simulink subsystem "PvtSubSys_VSM_ALL"  (R2020b)
settings: Solver=VariableStepAuto  StartTime=0.0  StopTime=10.0  RelTol=1e-3
values from neighbouring files (symbols this model uses):
  P_VSM_NOH_Act_Req = 0    [VSM_All.sldd]
  P_VSM_NOH_Swt_Req = 0    [VSM_All.sldd]
undefined symbols (not defined in the file or in its folder): ACC_STATE, HWA_STATE, LCK_STATE, P_VSM_ACCSOS_SW, P_VSM_AESSwtReq, P_VSM_CruiseFunUserInputMappingWays, P_VSM_ELKSwtReq, P_VSM_ESS_VehSwtReq, P_VSM_HWA_DMS_Enable, P_VSM_ICA_HandsOffSwtReq, P_VSM_IntelligentEvaSwtReq, P_VSM_ISLSwtReq, P_VSM_LCKSwtReq, P_VSM_LDWSwtReq, P_VSM_LKASwtReq, P_VSM_LSSSwtReq, P_VSM_PowerTrainConfig, P_VSM_SOSContinueTime, P_VSM_SOSSpdLimit, P_VSM_TSR_Dis_keep_SPL_Table, P_VSM_TSR_Dis_keep_SPLend, P_VSM_TSR_Dis_keep_TS_Table, P_VSM_TSR_Ena_SPLSupp_Table, P_VSM_TSR_Ena_TS_Table, P_VSM_TSR_SLIF_Speed_High, P_VSM_TSR_SLIF_Speed_Low, P_VSM_TSR_SLW_SnvtySwitch, P_VSM_TSR_SLW_Speed_Delta_disable, P_VSM_TSR_SLW_Speed_Delta_enable, P_VSM_TSR_SLW_Speed_High, P_VSM_TSR_SLW_Speed_Low, P_VSM_TSR_SLW_TrafEyeAvtiveDist, P_VSM_TSR_SLW_Warning_Time, P_VSM_TSR_SteerWheelAngle, P_VSM_TSR_SWS_speed_withDir, P_VSM_TSR_SWS_speed_woDir, P_VSM_TSRSwtReq, P_VSM_TSRWarnSwtReq, TJA_STATE, User_LC_ALCswt, User_LC_DrvConfirm, User_LC_DrvLCswt, User_LC_DrvOverride, User_LC_LeTurnNextLineReq, User_LC_RiTurnNextLineReq, User_LC_TurnMostLeLineReq, User_LC_TurnMostRiLineReq, User_LeTurnLmpOn, User_RiTurnLmpOn
libraries: simulink x51
(part 4 of 7)

== system PvtSubSys_VSM_ALL/Subsystem/StateManage/TSR2 ==
  note: Author:CZN
      | Version:V3.0
      | Data:20200919
      | Description:
      | 1.实现海外版TSR全部功能
      | Author:LC
      | Version:V3.1
      | Data:20200919
      | Description:
      | 1.新增掉头抑制条件判断；
      | 2.新增标定量P_VSM_TSR_SteerWheelAngle；
      | 3.新增观测量CAN输出
      | Author:LC
      | Version:V3.2
      | Data:20201008
      | Description:
      | 1.修复掉头抑制车速条件BUG；
      | Version:V3.3
      | Data:20201102
      | Description:
      | 1.修改超速报警抑制条件，从判断当前车速改为判断限速值；
      | 2.修改TSR_error条件下的状态跳转
      | 3.增加了灵敏度设置限幅；
      | 4.更改SLW_Enable信号来源；
      | 5.修复车速单位为英里时，报警值为公里数值问题；
      | 6.更改限速报警限速策略,改为融合发出信息就显示；
      | Version:V3.4
      | Data:20201103
      | Description:
      | 1、新增三个观测量；
      | 2、新增限速使能触发判断；
      | Version:V3.5
      | Data:20201105
      | Description:
      | 1、按照《交通标志信息功能规范》，新增仪表双位灯输出策略；
      | Version:V3.6
      | Data:20201201
      | Description:
      | 1、条件限速使能改为触发式；
  VehConfig : Inport
  Diag : Inport  Port=2
  RF_input : Inport  Port=3
  AD_CAN : Inport  Port=4
  HWAStateInfo : Inport  Port=5
  VSM_TSR_Init : Inport  Port=6
  Bus Creator : BusCreator  Inputs=25
  Bus Selector32 : BusSelector  OutputSignals=ISL_Active
  Bus Selector33 : BusSelector  OutputSignals=SPL_noSupp_Dist_Init,SPL_whSupp_Dist_Init,TS_SignName_Dist_Init,SPL_noSupp_Value_Init,SPL_whSupp_Value_Init,TS_SignName_Value_Init,SPL_SuppName_Value_Init
  Bus Selector6 : BusSelector  OutputSignals=FUSSts,RFframe_count,CtryType,RoadType,SPL_TypeCurRoad,SPL_ValueCurRoad,VehToTrafEyeDist,SPL_Unit,SPL_End,SPL_noSupp_Value,SPL_whSupp_Value,SPL_Sup1_SignName,SPL_Sup1_Confidence,SPL_Sup2_SignName,SPL_Sup2_Confidence,SPL_noSupp_LongDistance,SPL_whSupp_LongDistance,SPL_LeftLaneValue,SPL_RightLaneValue,TSR_ID,TS_SignName,TS_Confidence,TS_LongDistance,VehInLeftmostLane,VehInRightmostLane,SPL_LaneChanged
  Bus Selector7 : BusSelector  OutputSignals=TSRSwtReq,TSRWarnSwtReq,TSR_SnvtySet,SteerWheelAng,SteerWheelAngSign,VehSpd,IP_VehSpdUnit,RTurnLmpSwtSts,LTurnLmpSwtSts,VehYawRate,FFogLmpSts_F_Pbox,RFogLmpSts_R_Pbox,WindshldWiprActvSts,ACAmbTemp
  Bus Selector8 : BusSelector  OutputSignals=VehConfigTSR
  Bus Selector9 : BusSelector  OutputSignals=TSR_Error
  Data Type Conversion1 : DataTypeConversion
  Signal Conversion : SignalConversion  OverrideOpt=off
  Signal Conversion1 : SignalConversion  OverrideOpt=off
  TSRv3_4 : Subsystem
  TSR_output : Outport
  TSR_Measurements : Outport  Port=2
  wires:
  Bus Selector7/2 -> TSRv3_4/30(TSRWarnSwtReq)  "<TSRWarnSwtReq>"
  Bus Selector7/1 -> TSRv3_4/29(TSRSwtReq)  "<TSRSwtReq>"
  Bus Selector7/6 -> Data Type Conversion1/1  "<VehSpd>"
  Bus Selector6/23 -> TSRv3_4/25(TS_LongDistance)  "<TS_LongDistance>"
  TSRv3_4/25(TSDistKeep) -> Bus Creator/25
  TSRv3_4/26(TSR_Measurements) -> TSR_Measurements/1  "TSR_Measurements"
  VehConfig/1 -> Bus Selector8/1
  Bus Selector6/13 -> TSRv3_4/15(SPL_Sup1_Confidence)  "<SPL_Sup1_Confidence>"
  TSRv3_4/8(TSRSpdLimCfdc) -> Bus Creator/8
  TSRv3_4/6(TSRSpdLimSts) -> Bus Creator/6
  Bus Selector7/4 -> TSRv3_4/32(SteerWheelAng)  "<SteerWheelAng>"
  TSRv3_4/7(TSRSpdLim) -> Bus Creator/7
  TSRv3_4/14(SLW_Enable) -> Bus Creator/14
  TSRv3_4/9(TSRSpdLimWarn) -> Bus Creator/9
  Bus Selector6/18 -> TSRv3_4/20(SPL_LeftLaneValue)  "<SPL_LeftLaneValue>"
  Bus Selector6/6 -> TSRv3_4/8(SPL_ValueCurRoad)  "<SPL_ValueCurRoad>"
  Bus Selector33/1 -> TSRv3_4/44(SPL_noSupp_Dist_Init)  "<SPL_noSupp_Dist_Init>"
  Bus Selector33/4 -> TSRv3_4/47(SPL_noSupp_Value_Init)  "<SPL_noSupp_Value_Init>"
  Bus Selector6/9 -> TSRv3_4/11(SPL_End)  "<SPL_End>"
  Bus Selector7/3 -> TSRv3_4/31(TSR_SnvtySet)  "<TSR_SnvtySet>"
  Bus Selector9/1 -> TSRv3_4/2(TSR_error)  "<TSR_Error>"
  Bus Selector6/7 -> TSRv3_4/9(VehToTrafEyeDist)  "<VehToTrafEyeDist>"
  Bus Selector33/5 -> TSRv3_4/48(SPL_whSupp_Value_Init)  "<SPL_whSupp_Value_Init>"
  Bus Selector6/24 -> TSRv3_4/26(VehInLeftmostLane)  "<VehInLeftmostLane>"
  Bus Selector6/26 -> TSRv3_4/28(SPL_LaneChanged)  "<SPL_LaneChanged>"
  TSRv3_4/17(SPL_whSupp_Dist_Remain) -> Bus Creator/17
  Bus Selector7/11 -> TSRv3_4/39(FFogLmpSts_F_Pbox)  "<FFogLmpSts_F_Pbox>"
  Data Type Conversion1/1 -> TSRv3_4/34(VehSpd)
  Bus Selector6/4 -> TSRv3_4/6(RoadType)  "<RoadType>"
  Bus Selector7/9 -> TSRv3_4/37(LTurnLmpSwtSts)  "<LTurnLmpSwtSts>"
  TSRv3_4/5(TSRSpdLimUnit) -> Bus Creator/5
  Bus Selector7/10 -> TSRv3_4/38(VehYawRate)  "<VehYawRate>"
  TSRv3_4/22(SPL_SuppName_Value_Remain) -> Bus Creator/22
  TSRv3_4/13(TSRTrfcSignValCfdc) -> Bus Creator/13
  Bus Selector6/3 -> TSRv3_4/5(CtryType)  "<CtryType>"
  Bus Selector7/8 -> TSRv3_4/36(RTurnLmpSwtSts)  "<RTurnLmpSwtSts>"
  Bus Selector33/6 -> TSRv3_4/49(TS_SignName_Value_Init)  "<TS_SignName_Value_Init>"
  Bus Selector6/21 -> TSRv3_4/23(TS_SignName)  "<TS_SignName>"
  TSRv3_4/3(TSRWarnResp) -> Bus Creator/3
  TSRv3_4/12(TSRTrfcSignVal) -> Bus Creator/12
  Bus Selector7/13 -> TSRv3_4/41(WindshldWiprActvSts)  "<WindshldWiprActvSts>"
  Bus Selector6/11 -> Signal Conversion1/1  "<SPL_whSupp_Value>"
  Bus Selector6/1 -> TSRv3_4/3(FUSSts)  "<FUSSts>"
  Bus Selector6/16 -> TSRv3_4/18(SPL_noSupp_LongDistance)  "<SPL_noSupp_LongDistance>"
  TSRv3_4/2(TSRResp) -> Bus Creator/2
  Bus Selector6/8 -> TSRv3_4/10(SPL_Unit)  "<SPL_Unit>"
  TSRv3_4/24(SPLwhSuppDistKeep) -> Bus Creator/24
  Bus Selector8/1 -> TSRv3_4/1(VehConfigTSR)  "<VehConfigTSR>"
  Bus Selector7/14 -> TSRv3_4/42(ACAmbTemp)  "<ACAmbTemp>"
  TSRv3_4/10(TSRConSpdLim) -> Bus Creator/10
  Bus Selector32/1 -> TSRv3_4/43(ISLActive_sts)  "<ISL_Active>"
  Bus Selector7/12 -> TSRv3_4/40(RFogLmpSts_R_Pbox)  "<RFogLmpSts_R_Pbox>"
  Bus Selector6/25 -> TSRv3_4/27(VehInRightmostLane)  "<VehInRightmostLane>"
  TSRv3_4/1(TSRSts) -> Bus Creator/1
  TSRv3_4/11(TSRConSpdLimWarn) -> Bus Creator/11
  Bus Selector7/7 -> TSRv3_4/35(IP_VehSpdUnit)  "<IP_VehSpdUnit>"
  TSRv3_4/19(SPL_noSupp_Value_Remain) -> Bus Creator/19
  Bus Selector6/2 -> TSRv3_4/4(RFframe_count)  "<RFframe_count>"
  Bus Selector6/20 -> TSRv3_4/22(TSR_ID)  "<TSR_ID>"
  Bus Selector33/7 -> TSRv3_4/50(SPL_SuppName_Value_Init)  "<SPL_SuppName_Value_Init>"
  Bus Selector6/10 -> Signal Conversion/1  "<SPL_noSupp_Value>"
  TSRv3_4/4(TSR_Snvty) -> Bus Creator/4
  TSRv3_4/18(TS_SignName_Dist_Remain) -> Bus Creator/18
  TSRv3_4/21(TS_SignName_Value_Remain) -> Bus Creator/21
  TSRv3_4/15(SLW_SpeedLimitValueWhSnvty) -> Bus Creator/15
  TSRv3_4/23(SPLnoSuppDistKeep) -> Bus Creator/23
  TSRv3_4/16(SPL_noSupp_Dist_Remain) -> Bus Creator/16
  Bus Selector6/5 -> TSRv3_4/7(SPL_TypeCurRoad)  "<SPL_TypeCurRoad>"
  Bus Selector6/22 -> TSRv3_4/24(TS_Confidence)  "<TS_Confidence>"
  Bus Selector33/3 -> TSRv3_4/46(TS_SignName_Dist_Init)  "<TS_SignName_Dist_Init>"
  Bus Selector33/2 -> TSRv3_4/45(SPL_whSupp_Dist_Init)  "<SPL_whSupp_Dist_Init>"
  Bus Selector6/14 -> TSRv3_4/16(SPL_Sup2_SignName)  "<SPL_Sup2_SignName>"
  Bus Selector7/5 -> TSRv3_4/33(SteerWheelAngSign)  "<SteerWheelAngSign>"
  Bus Selector6/19 -> TSRv3_4/21(SPL_RightLaneValue)  "<SPL_RightLaneValue>"
  Bus Selector6/15 -> TSRv3_4/17(SPL_Sup2_Confidence)  "<SPL_Sup2_Confidence>"
  Bus Selector6/17 -> TSRv3_4/19(SPL_whSupp_LongDistance)  "<SPL_whSupp_LongDistance>"
  Bus Selector6/12 -> TSRv3_4/14(SPL_Sup1_SignName)  "<SPL_Sup1_SignName>"
  TSRv3_4/20(SPL_whSupp_Value_Remain) -> Bus Creator/20
  HWAStateInfo/1 -> Bus Selector32/1
  RF_input/1 -> Bus Selector6/1
  AD_CAN/1 -> Bus Selector7/1
  Diag/1 -> Bus Selector9/1
  VSM_TSR_Init/1 -> Bus Selector33/1
  Bus Creator/1 -> TSR_output/1  "TSR_output"
  Signal Conversion/1 -> TSRv3_4/12(SPL_noSupp_Value)
  Signal Conversion1/1 -> TSRv3_4/13(SPL_whSupp_Value)

== system PvtSubSys_VSM_ALL/Subsystem/StateManage/UOM ==
  CSA : Inport
  FunFeedBack : Inport  Port=2
  Constant : Constant  Value=P_VSM_CruiseFunUserInputMappingWays
  GW_V71 : Subsystem
  Terminator : Terminator
  UserOperation : Outport
  wires:
  Constant/1 -> Terminator/1
  CSA/1 -> GW_V71/1(AD)
  FunFeedBack/1 -> GW_V71/2(FunFeedback)
  GW_V71/1(UserOperation) -> UserOperation/1  "UserOperation"

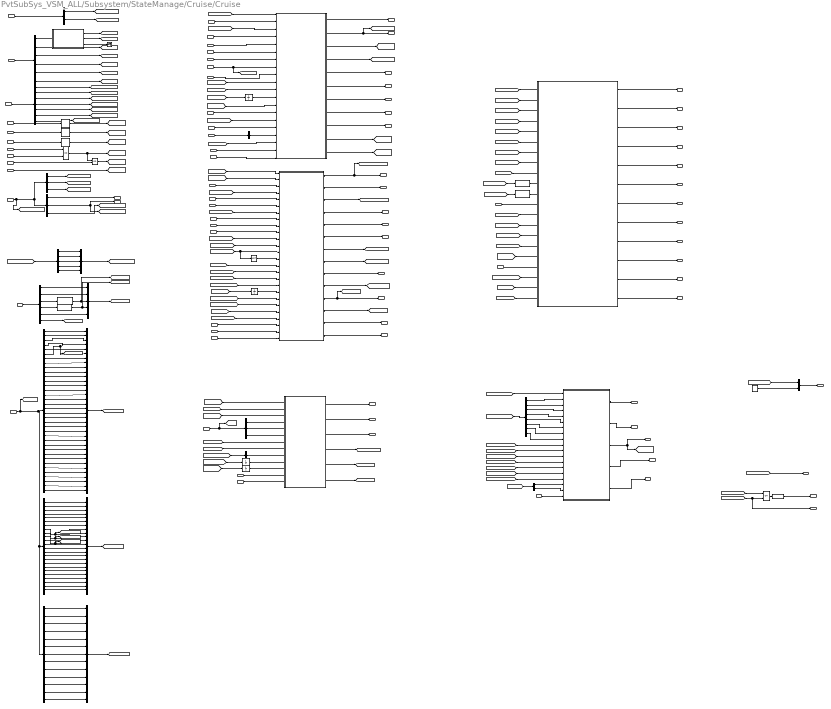
== system PvtSubSys_VSM_ALL/Subsystem/StateManage/Cruise/Cruise ==
  ACCError : Inport  OutDataTypeStr=uint8
  HWAError : Inport  Port=2  OutDataTypeStr=uint8
  "\tTJAError" : Inport  Port=3
  VehConfigHWA : Inport  Port=4  OutDataTypeStr=uint8
  VehConfigTJA : Inport  Port=5  OutDataTypeStr=uint8
  VehConfigACC : Inport  Port=6  OutDataTypeStr=uint8
  VehConfigiACC : Inport  Port=7  OutDataTypeStr=uint8
  ObjFailure_b : Inport  Port=8
  TargetExist_b : Inport  Port=9
  <dxP0> : Inport  Port=10
  axvRefMs2 : Inport  Port=11
  VxvRef_ms : Inport  Port=12
  DriveOffConditonFulfilled_b : Inport  Port=13
  AEB_Trigger : Inport  Port=14
  Longctrl_Decel_ReqValue : Inport  Port=15
  LCK_State : Inport  Port=16
  TJA_LCKState : Inport  Port=17
  DoubleLineLost_b : Inport  Port=18
  HWALineValid : Inport  Port=19
  TJALineValid : Inport  Port=20
  AD_CAN : Inport  Port=21
  DriverSts : Inport  Port=22
  TSR_output : Inport  Port=23
  DirverOperation : Inport  Port=24
  HODinfo : Inport  Port=25
  ALC : Inport  Port=26
  VSM_ESSState : Inport  Port=27
  PilotSts : Inport  Port=28
  EHR_Input : Inport  Port=29
  PLAN_NOH_SetSpdAdjReq : Inport  Port=30
  PLAN_NOH_SetSpdAdjVal : Inport  Port=31
  LSM_PilotNohExitDist : Inport  Port=32
  TimeGapInit : Inport  Port=33
  IB_BrkPedalAppld : Inport  Port=34
  ConfigiBooster : Inport  Port=35
  ACC : Subsystem  ReferencedSubsystem=PvtSubSys_VSM_ACC
  ACC_AD : BusCreator  Inputs=36
  AD_CAN1 : InportShadow  Port=21
  AD_CAN2 : InportShadow  Port=21
  AEB_Trigger1 : InportShadow  Port=14
  Bus Creator3 : BusCreator  Inputs=2
  Bus Creator4 : BusCreator  Inputs=5
  Bus Creator8 : BusCreator  Inputs=5
  Bus Selector : BusSelector  OutputSignals=NavRoadType
  Bus Selector1 : BusSelector  OutputSignals=SLW_SpdLimValue,SLW_Enable,TSRWarnResp
  Bus Selector10 : BusSelector  OutputSignals=AccelPedlPosnDiagc,ESP_MasterCylBrkPress,BrkPedalSts,EPBSts,EPB_SwtPosn,VehStandstill,RLWheelSpd,RRWheelSpd,RLWheelDriveDirection,RRWheelDriveDirection,TGS_LEVER,EngState,Start_StopSts,ESPFuncOffSts,BrkDskOvrheatd,DrvDoorSts,DrvSBR,CC_ACC_CANCEL_OFFSwt,VDCActv,MSRActv,HDCCtrl,ABSActv,PTCActv,BTCActv,AVHSts,VehSpd,AccPedalOverride,DrivingModDis,EngLimpHomeSts,APS_WorkSts,ECMACCInterface,CDDAvailable,SysPowerMod,CDDActv,HCU_PowertrainSts,HCU_GearSts
  Bus Selector11 : BusSelector  OutputSignals=User_DecSetSpd_S,User_DecSetSpd_L,User_IncSetSpd_S,User_IncSetSpd_L,VSM_User_ACCSet,User_TimeGapDec,User_TimeGapInc,VSM_User_ACCRes
  Bus Selector12 : BusSelector  OutputSignals=VehSpd,IP_VehSpdUnit,TGS_LEVER,CDDActv,ISLSwtReq,TSRSwtReq
  Bus Selector13 : BusSelector  OutputSignals=USS_FrontSys_Status,USS_FLCNear_Obj_Confidence,USS_FLCNear_Obj_Pos_X,USS_FLCNear_Obj_Pos_Y,USS_FLMNear_Obj_Confidence,USS_FLMNear_Obj_Pos_X,USS_FLMNear_Obj_Pos_Y,USS_FRMNear_Obj_Confidence,USS_FRMNear_Obj_Pos_X,USS_FRMNear_Obj_Pos_Y,USS_FRCNear_Obj_Confidence,USS_FRCNear_Obj_Pos_X,USS_FRCNear_Obj_Pos_Y
  Bus Selector14 : BusSelector  OutputSignals=DrvSBR,PassSBR
  Bus Selector2 : BusSelector  OutputSignals=ACCon,TJAOn,VSM_User_ACCSet,VSM_User_ACCRes,VSM_User_TJASet
  Bus Selector3 : BusSelector  OutputSignals=TJA_ACC_SelSts,TJAOn,HWA_Swt
  Bus Selector4 : BusSelector  OutputSignals=User_ISLSet
  Bus Selector5 : BusSelector  OutputSignals=PLAN_ALC_LcDecsLe,PLAN_ALC_LcDecsRi,PLAN_ALC_TurnLightReq,PLAN_ALC_LcFeReason,PLAN_ALC_sts,PLAN_ALC_LcCancelReason,PLAN_ALC_stsReason
  Bus Selector6 : BusSelector  OutputSignals=signal1.DrivingOnHighWay,signal1.FormOfWay,signal1.TunnelDistance,signal1.RampDistance,MapDataValid,signal1.i_road_curvature_far
  Bus Selector7 : BusSelector  OutputSignals=HandsOffWarnLevel,HandsOffDetd
  Bus Selector8 : BusSelector  OutputSignals=DVRWorkSts,VDCActv,MSRActv,HDCCtrl,ABSActv,PTCActv,BTCActv,LTurnLmpSwtSts,RTurnLmpSwtSts,HazardLmpSwtSts,EPBSts,EPB_SwtPosn,VehStandstill,TGS_LEVER,ESPFuncOffSts,DrvDoorSts,DrvSBR,VehSpd,ESP_MasterCylBrkPress,BrkPedalSts,NOH_Swt_Req,NOH_Act_Req,HCU_GearSts,PassSBR
  Bus Selector9 : BusSelector  OutputSignals=VSM_User_ACCSet,VSM_User_ACCRes,VSM_User_TJASet
  Constant : Constant  Value=false
  Data Type Conversion : DataTypeConversion
  Data Type Conversion1 : DataTypeConversion
  Data Type Conversion2 : DataTypeConversion  OutDataTypeStr=double
  Data Type Conversion3 : DataTypeConversion  OutDataTypeStr=uint16
  Data Type Conversion4 : DataTypeConversion  OutDataTypeStr=uint16
  DriverSts1 : InportShadow  Port=22
  DriverSts2 : InportShadow  Port=22
  HWA : Subsystem  ReferencedSubsystem=PvtSubSys_VSM_HWA
  HWA_AD : BusCreator  Inputs=24
  HWA_AD1 : BusCreator  Inputs=13
  ISL : Subsystem  ReferencedSubsystem=PvtSubSys_VSM_ISL
  LngHMI : Subsystem  ReferencedSubsystem=PvtSubSys_VSM_LngHMI
  Logical Operator : Logic  Operator=NOT  AllPortsSameDT=off  OutDataTypeStr=boolean
  Logical Operator2 : Logic  Operator=OR  AllPortsSameDT=off  OutDataTypeStr=boolean
  Logical Operator3 : Logic  Operator=OR  AllPortsSameDT=off  OutDataTypeStr=boolean
  Logical Operator4 : Logic  Operator=OR  AllPortsSameDT=off  OutDataTypeStr=boolean
  SetSpd : Subsystem  ReferencedSubsystem=PvtSubSys_VSM_SetSpd
  Signal Conversion : SignalConversion  OverrideOpt=off
  Signal Conversion1 : SignalConversion  OverrideOpt=off
  Signal Conversion2 : SignalConversion  OverrideOpt=off
  Terminator1 : Terminator
  Unit Delay : UnitDelay  SampleTime=-1  HasFrameUpgradeWarning=on
  Unit Delay1 : UnitDelay  SampleTime=-1  HasFrameUpgradeWarning=on
  Unit Delay3 : UnitDelay  InitialCondition=ACC_STATE.ACC_Off  SampleTime=-1  HasFrameUpgradeWarning=on
  Unit Delay4 : UnitDelay  SampleTime=-1  HasFrameUpgradeWarning=on
  VehSpdCalc : Subsystem
  HWA_LaneChangeReq : Outport
  Signal_ACC_SpdSetValue : Outport  Port=2
  Signal_ACC_HazActv : Outport  Port=3
  Signal_ACC_TimeGapSet : Outport  Port=4
  Signal_ACC_DrvOFF_Req : Outport  Port=5
  vSetBelowMin : Outport  Port=6
  Signal_ACC_ModDisp : Outport  Port=7
  Signal_TJA_ACC_SelSts : Outport  Port=8
  TJA_ON : Outport  Port=9  OutDataTypeStr=boolean
  Signal_ACC_ModeSts : Outport  Port=10
  ACCParkShiftReq : Outport  Port=11
  Signal_TJA_ModeSts : Outport  Port=12
  Signal_CruiseChauffer_Sts : Outport  Port=13
  Signal_ACCTextDisp : Outport  Port=14
  Signal_TJATextDisp : Outport  Port=15
  Signal_CCTextDisp : Outport  Port=16
  HWASts : Outport  Port=17
  TJASts : Outport  Port=18
  HWAActive : Outport  Port=19
  HWAWarningLevel : Outport  Port=20
  Signal_HWAModeDisp : Outport  Port=21
  ISL_Resp : Outport  Port=22
  ISL_InterSysInfoDisp : Outport  Port=23
  ISLActive : Outport  Port=24
  SetSpeedKmh : Outport  Port=25
  Signal_HWATextDisp : Outport  Port=26
  Signal_DriverOffDisp : Outport  Port=27
  Signal_NOH_Sts : Outport  Port=28
  Signal_NOH_SysInfoDisplay : Outport  Port=29
  Signal_NOH_DistToExit : Outport  Port=30
  HWAParkShiftReq : Outport  Port=31
  EDR_DriverBrakeHWAExit : Outport  Port=32
  EDR_OverrideHWAExit : Outport  Port=33
  UOMSysFeedBack : Outport  Port=34
  ACCDataClct_ConNotStsf : Outport  Port=35
  ACCDataClct_OverrideACCExit : Outport  Port=36
  ACCDataClct_DriverBrakeACCExit : Outport  Port=37
  ACCDataClct_DriverSteerACCExit : Outport  Port=38
  TJADataClct_ConNotStsf : Outport  Port=39
  HWA_TurnLightReq : Outport  Port=40
  NOHActiveNum : Outport  Port=41
  ACC_TimeGapSetHMI : Outport  Port=42
  wires:
  Bus Selector11/8 -> SetSpd/9  "<VSM_User_ACCRes>"
  Bus Selector8/24 -> HWA_AD/24  "<PassSBR>"
  Bus Selector8/23 -> HWA_AD/23  "<HCU_GearSts>"
  [i_road_curvature_far] -> LngHMI/21
  Bus Selector6/6 -> [i_road_curvature_far]  "<i_road_curvature_far>"
  ConfigiBooster/1 -> ACC/20
  IB_BrkPedalAppld/1 -> ACC/19
  [AEB_Trigger] -> LngHMI/20
  TimeGapInit/1 -> SetSpd/19
  SetSpd/5 -> ACC_TimeGapSetHMI/1
  Bus Selector10/36 -> ACC_AD/36  "<HCU_GearSts>"
  Bus Selector10/35 -> ACC_AD/35  "<HCU_PowertrainSts>"
  HWA/14 -> NOHActiveNum/1
  Bus Selector8/22 -> HWA_AD/22  "<NOH_Act_Req>"
  HWA/13 -> Signal_NOH_Sts/1
  [TJAError] -> HWA/2
  Signal Conversion2/1 -> [TJAError]  "VSM_Diagnostic_TJAError"
  "\tTJAError"/1 -> Signal Conversion2/1
  [TJASts] -> ACC/18
  TJA_LCKState/1 -> HWA/25
  VSM_ESSState/1 -> HWA/24
  [Switch_SetTJA] -> HWA/23
  [VehConfigTJA] -> HWA/22
  [PLAN_ALC_sts] -> HWA/21
  [PLAN_ALC_LcFeReason] -> HWA/20
  Unit Delay/1 -> HWA/19
  [PLAN_ALC_TurnLightReq] -> HWA/18
  [PLAN_ALC_LeTurnReq] -> HWA/17
  [PLAN_ALC_RiTurnReq] -> HWA/16
  Logical Operator/1 -> HWA/14
  [HandsOffWarningLevel] -> HWA/12
  [HWA_AD_CAN] -> HWA/11
  LCK_State/1 -> HWA/10
  DriverSts1/1 -> HWA/9
  PilotSts/1 -> HWA/8
  [EHR_bus] -> HWA/7
  HWALineValid/1 -> HWA/6
  [ACCSts] -> HWA/4
  DoubleLineLost_b/1 -> HWA/5
  AEB_Trigger/1 -> HWA/3
  <dxP0>/1 -> ACC/16
  DriverSts2/1 -> ACC/14
  [ACCError] -> ACC/13
  [HAP_CAN] -> ACC/15
  Bus Selector/1 -> ACC/17  "<NavRoadType>"
  [VehConfigACC] -> ACC/11
  [VehConfigTJA] -> ACC/10
  ObjFailure_b/1 -> ACC/9
  AEB_Trigger1/1 -> ACC/8, [AEB_Trigger]
  ACC/11 -> [ACCFailure]
  ACC/10 -> [DrvrOff_Disp]
  ACC/9 -> TJADataClct_ConNotStsf/1
  ACC/8 -> ACCDataClct_DriverSteerACCExit/1
  ACC/7 -> ACCDataClct_DriverBrakeACCExit/1
  ACC/6 -> ACCDataClct_OverrideACCExit/1
  ACC/5 -> ACCDataClct_ConNotStsf/1
  ACC/4 -> [ACC_DriverCancel]
  ACC/3 -> [AccOverride]
  ACC/2 -> [ACCSts], Signal_ACC_ModeSts/1
  HWA/10 -> [TJASafeStopExit_b]
  HWA/11 -> TJASts/1, [TJASts]
  HWA/9 -> HWA_TurnLightReq/1
  HWA/8 -> [VSM_HWANOA_Mode]
  HWA/7 -> [HWAWarningLevel]
  HWA/3 -> [HWAParkShift]
  HWA/4 -> HWA_LaneChangeReq/1
  HWA/6 -> EDR_OverrideHWAExit/1
  HWA/5 -> EDR_DriverBrakeHWAExit/1
  TJALineValid/1 -> HWA/26
  Bus Selector3/3 -> [HWASwt]  "<HWA_Swt>"
  [PLAN_ALC_stsReason] -> LngHMI/19
  Bus Selector5/7 -> [PLAN_ALC_stsReason]  "<PLAN_ALC_stsReason>"
  Bus Selector5/6 -> [PLAN_ALC_LcCancelReason]  "<PLAN_ALC_LcCancelReason>"
  Bus Selector5/5 -> [PLAN_ALC_sts]  "<PLAN_ALC_sts>"
  Bus Selector5/4 -> [PLAN_ALC_LcFeReason]  "<PLAN_ALC_LcFeReason>"
  LngHMI/12 -> Signal_NOH_DistToExit/1  "VSM_NOH_DistToExit"
  LngHMI/11 -> Signal_NOH_SysInfoDisplay/1  "VSM_NOH_SysInfoDisplay"
  LSM_PilotNohExitDist/1 -> LngHMI/18
  LngHMI/10 -> Signal_DriverOffDisp/1  "ACC_DrvrOffDisp"
  AD_CAN2/1 -> Bus Selector/1
  [TSRSwtReq] -> ISL/2
  Bus Selector12/6 -> [TSRSwtReq]  "<TSRSwtReq>"
  HWA_AD1/1 -> [HAP_CAN]
  Bus Selector13/13 -> HWA_AD1/13  "<USS_FRCNear_Obj_Pos_Y>"
  Bus Selector13/12 -> HWA_AD1/12  "<USS_FRCNear_Obj_Pos_X>"
  Bus Selector13/11 -> HWA_AD1/11  "<USS_FRCNear_Obj_Confidence>"
  Bus Selector13/10 -> HWA_AD1/10  "<USS_FRMNear_Obj_Pos_Y>"
  Bus Selector13/9 -> HWA_AD1/9  "<USS_FRMNear_Obj_Pos_X>"
  Bus Selector13/8 -> HWA_AD1/8  "<USS_FRMNear_Obj_Confidence>"
  Bus Selector13/7 -> HWA_AD1/7  "<USS_FLMNear_Obj_Pos_Y>"
  Bus Selector13/6 -> HWA_AD1/6  "<USS_FLMNear_Obj_Pos_X>"
  Bus Selector13/5 -> HWA_AD1/5  "<USS_FLMNear_Obj_Confidence>"
  Bus Selector13/4 -> HWA_AD1/4  "<USS_FLCNear_Obj_Pos_Y>"
  Bus Selector13/3 -> HWA_AD1/3  "<USS_FLCNear_Obj_Pos_X>"
  Bus Selector13/2 -> HWA_AD1/2  "<USS_FLCNear_Obj_Confidence>"
  Bus Selector13/1 -> HWA_AD1/1  "<USS_FrontSys_Status>"
  PLAN_NOH_SetSpdAdjVal/1 -> ISL/13
  PLAN_NOH_SetSpdAdjReq/1 -> ISL/12
  [DrvrOff_Disp] -> LngHMI/17
  [VSM_HWANOA_Mode] -> LngHMI/16
  Bus Selector5/3 -> [PLAN_ALC_TurnLightReq]  "<PLAN_ALC_TurnLightReq>"
  Data Type Conversion4/1 -> Bus Creator4/4, [RampDistance]  "RampDistance"
  Data Type Conversion3/1 -> Bus Creator4/3, [TunnelDistance]  "TunnelDistance"
  Data Type Conversion1/1 -> LngHMI/11
  Data Type Conversion/1 -> LngHMI/10
  Bus Selector11/1 -> SetSpd/2  "<User_DecSetSpd_S>"
  Bus Selector11/2 -> SetSpd/3  "<User_DecSetSpd_L>"
  Bus Selector11/7 -> SetSpd/8  "<User_TimeGapInc>"
  Bus Selector11/3 -> SetSpd/4  "<User_IncSetSpd_S>"
  Bus Selector11/6 -> SetSpd/7  "<User_TimeGapDec>"
  Bus Selector11/4 -> SetSpd/5  "<User_IncSetSpd_L>"
  Bus Selector11/5 -> SetSpd/6  "<VSM_User_ACCSet>"
  [Switch_SetTJA] -> LngHMI/15
  [Switch_Set] -> LngHMI/14
  [Switch_Res] -> LngHMI/13
  DriverSts/1 -> LngHMI/12
  [RampDistance] -> Data Type Conversion1/1
  [TunnelDistance] -> Data Type Conversion/1
  Bus Selector9/1 -> [Switch_Set]  "<VSM_User_ACCSet>"
  Bus Selector9/3 -> [Switch_SetTJA]  "<VSM_User_TJASet>"
  Bus Selector9/2 -> [Switch_Res]  "<VSM_User_ACCRes>"
  Bus Selector5/2 -> [PLAN_ALC_RiTurnReq]  "<PLAN_ALC_LcDecsRi>"
  Bus Selector5/1 -> [PLAN_ALC_LeTurnReq]  "<PLAN_ALC_LcDecsLe>"
  ALC/1 -> Bus Selector5/1
  [TJA_ON] -> HWA/15
  [HandsOff_b] -> HWA/13, Logical Operator/1
  [HWAError] -> HWA/1
  HWA/2 -> HWAActive/1
  HWA/1 -> [HWASts], HWASts/1
  Bus Selector10/34 -> ACC_AD/34  "<CDDActv>"
  [ACC_DirverOperation] -> ACC/1
  ACC/1 -> Signal_ACC_DrvOFF_Req/1
  Longctrl_Decel_ReqValue/1 -> ACC/7
  VxvRef_ms/1 -> ACC/6
  axvRefMs2/1 -> ACC/5
  TargetExist_b/1 -> ACC/4
  [ACC_AD_CAN] -> ACC/3
  DriveOffConditonFulfilled_b/1 -> ACC/2
  Bus Selector12/5 -> [ISLSwtReq]  "<ISLSwtReq>"
  Bus Selector12/4 -> [CDDActv]  "<CDDActv>"
  Bus Selector12/3 -> [TGS_LEVER]  "<TGS_LEVER>"
  Bus Selector12/2 -> [IP_VehSpdUnit]  "<IP_VehSpdUnit>"
  AD_CAN1/1 -> Bus Selector12/1
  Bus Selector8/1 -> HWA_AD/1  "<DVRWorkSts>"
  [VehSpdIPmph] -> SetSpd/16
  [VehSpdIP] -> SetSpd/15
  [ACCSts] -> SetSpd/12
  [TJASts] -> SetSpd/13
  [HWASts] -> SetSpd/14
  [ISL_SetSpdAdjVal] -> SetSpd/11
  [DirverOperation] -> Bus Selector11/1
  Bus Creator8/1 -> [ACC_DirverOperation]
  Bus Selector2/1 -> Bus Creator8/1  "<ACCon>"
  Bus Selector2/5 -> Bus Creator8/5  "<VSM_User_TJASet>"
  Bus Selector2/2 -> Bus Creator8/2  "<TJAOn>"
  Bus Selector2/4 -> Bus Creator8/4  "<VSM_User_ACCRes>"
  Bus Selector2/3 -> Bus Creator8/3  "<VSM_User_ACCSet>"
  [HWAParkShift] -> Logical Operator4/2, HWAParkShiftReq/1
  Logical Operator4/1 -> Data Type Conversion2/1
  [ACC_ParkShiftReq] -> Logical Operator4/1
  [ISL_SetSpdAdjReq] -> SetSpd/10
  [IP_VehSpdUnit] -> SetSpd/1
  ACC_AD/1 -> [ACC_AD_CAN]
  Bus Selector10/33 -> ACC_AD/33  "<SysPowerMod>"
  Bus Selector10/32 -> ACC_AD/32  "<CDDAvailable>"
  Bus Selector10/31 -> ACC_AD/31  "<ECMACCInterface>"
  Bus Selector10/30 -> ACC_AD/30  "<APS_WorkSts>"
  Bus Selector10/29 -> ACC_AD/29  "<EngLimpHomeSts>"
  Bus Selector10/28 -> ACC_AD/28  "<DrivingModDis>"
  Bus Selector10/27 -> ACC_AD/27  "<AccPedalOverride>"
  Bus Selector10/26 -> ACC_AD/26  "<VehSpd>"
  Bus Selector10/25 -> ACC_AD/25  "<AVHSts>"
  Bus Selector10/24 -> ACC_AD/24  "<BTCActv>"
  Bus Selector10/23 -> ACC_AD/23  "<PTCActv>"
  Bus Selector10/1 -> ACC_AD/1  "<AccelPedlPosnDiagc>"
  Bus Selector10/22 -> ACC_AD/22  "<ABSActv>"
  Bus Selector10/2 -> ACC_AD/2  "<ESP_MasterCylBrkPress>"
  Bus Selector10/21 -> ACC_AD/21  "<HDCCtrl>"
  Bus Selector10/3 -> ACC_AD/3  "<BrkPedalSts>"
  Bus Selector10/20 -> ACC_AD/20  "<MSRActv>"
  Bus Selector10/4 -> ACC_AD/4  "<EPBSts>"
  Bus Selector10/19 -> ACC_AD/19  "<VDCActv>"
  Bus Selector10/5 -> ACC_AD/5  "<EPB_SwtPosn>"
  Bus Selector10/18 -> ACC_AD/18  "<CC_ACC_CANCEL_OFFSwt>"
  Bus Selector10/6 -> ACC_AD/6, [VehicleStandstill]  "<VehStandstill>"
  Bus Selector10/17 -> ACC_AD/17  "<DrvSBR>"
  Bus Selector10/7 -> ACC_AD/7  "<RLWheelSpd>"
  Bus Selector10/16 -> ACC_AD/16  "<DrvDoorSts>"
  Bus Selector10/8 -> ACC_AD/8  "<RRWheelSpd>"
  Bus Selector10/15 -> ACC_AD/15  "<BrkDskOvrheatd>"
  Bus Selector10/9 -> ACC_AD/9  "<RLWheelDriveDirection>"
  Bus Selector10/14 -> ACC_AD/14  "<ESPFuncOffSts>"
  Bus Selector10/10 -> ACC_AD/10  "<RRWheelDriveDirection>"
  Bus Selector10/13 -> ACC_AD/13  "<Start_StopSts>"
  Bus Selector10/11 -> ACC_AD/11  "<TGS_LEVER>"
  Bus Selector10/12 -> ACC_AD/12  "<EngState>"
  HWA_AD/1 -> [HWA_AD_CAN]
  Bus Selector8/20 -> HWA_AD/20  "<BrkPedalSts>"
  Bus Selector8/19 -> HWA_AD/19  "<ESP_MasterCylBrkPress>"
  Bus Selector8/2 -> HWA_AD/2  "<VDCActv>"
  Bus Selector8/18 -> HWA_AD/18  "<VehSpd>"
  Bus Selector8/3 -> HWA_AD/3  "<MSRActv>"
  Bus Selector8/17 -> HWA_AD/17  "<DrvSBR>"
  Bus Selector8/4 -> HWA_AD/4  "<HDCCtrl>"
  Bus Selector8/16 -> HWA_AD/16  "<DrvDoorSts>"
  Bus Selector8/5 -> HWA_AD/5  "<ABSActv>"
  Bus Selector8/15 -> HWA_AD/15  "<ESPFuncOffSts>"
  Bus Selector8/6 -> HWA_AD/6  "<PTCActv>"
  Bus Selector8/14 -> HWA_AD/14  "<TGS_LEVER>"
  Bus Selector8/7 -> HWA_AD/7  "<BTCActv>"
  Bus Selector8/13 -> HWA_AD/13  "<VehStandstill>"
  Bus Selector8/8 -> HWA_AD/8, [LTurnLmpSwtSts]  "<LTurnLmpSwtSts>"
  Bus Selector8/12 -> HWA_AD/12  "<EPB_SwtPosn>"
  Bus Selector8/9 -> HWA_AD/9, [RTurnLmpSwtSts]  "<RTurnLmpSwtSts>"
  Bus Selector8/11 -> HWA_AD/11  "<EPBSts>"
  Bus Selector8/10 -> HWA_AD/10, [HazardLmpSwtSts]  "<HazardLmpSwtSts>"
  AD_CAN/1 -> [AD_CAN], Bus Selector10/1, Bus Selector8/1, Bus Selector13/1
  Bus Creator4/1 -> [EHR_bus]
  Bus Selector6/5 -> Bus Creator4/5  "<MapDataValid>"
  Bus Selector6/4 -> Data Type Conversion4/1  "<RampDistance>"
  Bus Selector6/3 -> Data Type Conversion3/1  "<TunnelDistance>"
  Bus Selector6/2 -> Bus Creator4/2  "<FormOfWay>"
  Bus Selector6/1 -> Bus Creator4/1  "<DrivingOnHighWay>"
  EHR_Input/1 -> Bus Selector6/1
  SetSpd/2 -> vSetBelowMin/1  "vSetBelowMin"
  SetSpd/4 -> Signal_ACC_SpdSetValue/1  "Signal_ACC_SpdSetValue"
  SetSpd/1 -> Signal_ACC_TimeGapSet/1  "Signal_ACC_TimeGapSet"
  Bus Selector3/1 -> Signal_TJA_ACC_SelSts/1  "<TJA_ACC_SelSts>"
  Data Type Conversion2/1 -> ACCParkShiftReq/1  "Signal_ACC_ParkShiftReq"
  [HWAWarningLevel] -> HWAWarningLevel/1
  Bus Selector1/1 -> ISL/4  "<SLW_SpdLimValue>"
  Bus Selector1/2 -> ISL/5  "<SLW_Enable>"
  [ISLSwtReq] -> ISL/3
  ISL/1 -> ISL_Resp/1  "ISL_Resp"
  ISL/3 -> ISL_InterSysInfoDisp/1
  ISL/2 -> ISLActive/1
  ISL/4 -> [ISL_ReqUserConfirm]
  TSR_output/1 -> Bus Selector1/1, [TSRinfo]
  VehConfigHWA/1 -> Logical Operator2/1
  VehConfigTJA/1 -> Logical Operator2/2
  VehConfigiACC/1 -> [VehConfigiACC]
  VehConfigACC/1 -> Logical Operator3/2
  Logical Operator2/1 -> [VehConfigTJA], Logical Operator3/1
  Logical Operator3/1 -> [VehConfigACC]
  Signal Conversion/1 -> [ACCError]  "VSM_Diagnostic_ACCError"
  Signal Conversion1/1 -> [HWAError]  "VSM_Diagnostic_HWAError"
  Bus Selector1/3 -> ISL/6  "<TSRWarnResp>"
  [TJASts] -> ISL/7
  [HWASts] -> ISL/8
  ISL/6 -> [ISL_SetSpdAdjVal]
  [DirverOperation] -> Bus Selector2/1
  DirverOperation/1 -> Bus Selector9/1, Bus Selector3/1, [DirverOperation]
  Bus Selector3/2 -> [TJA_ON], TJA_ON/1  "<TJAOn>"
  [DirverOperation] -> Bus Selector4/1
  Bus Selector4/1 -> ISL/9  "<User_ISLSet>"
  [VehConfigiACC] -> ISL/1
  SetSpd/3 -> SetSpeedKmh/1, [SetSpeedKmH]  "SetSpeedKmH"
  [ACCSts] -> Unit Delay3/1
  [SetSpeedKmH] -> Unit Delay4/1
  ACCError/1 -> Signal Conversion/1
  HWAError/1 -> Signal Conversion1/1
  HODinfo/1 -> Bus Selector7/1
  Bus Selector7/1 -> [HandsOffWarningLevel]  "<HandsOffWarnLevel>"
  Bus Selector7/2 -> [HandsOff_b]  "<HandsOffDetd>"
  Bus Selector12/1 -> VehSpdCalc/1(VehicleSpd)  "<VehSpd>"
  VehSpdCalc/1(IP_VehSpd_kmh) -> [VehSpdIP]
  VehSpdCalc/3(ESP_VehSpd_kmh) -> Terminator1/1
  VehSpdCalc/2(IP_VehSpd_mph) -> [VehSpdIPmph]
  Unit Delay3/1 -> ISL/10
  Unit Delay4/1 -> ISL/11
  ISL/5 -> [ISL_SetSpdAdjReq]
  [HWAWarningLevel] -> LngHMI/1
  [HandsOffWarningLevel] -> LngHMI/2
  [HazardLmpSwtSts] -> LngHMI/3
  [ACCSts] -> LngHMI/5
  [ACC_DriverCancel] -> LngHMI/4
  [TJASts] -> LngHMI/6
  [HWASts] -> LngHMI/7
  [TJASafeStopExit_b] -> LngHMI/8
  [VehicleStandstill] -> LngHMI/9
  LngHMI/1 -> Signal_ACC_HazActv/1  "Signal_ACC_HazActv"
  LngHMI/2 -> Signal_ACC_ModDisp/1  "Signal_ACC_ModDisp"
  LngHMI/3 -> Signal_TJA_ModeSts/1  "Signal_TJA_ModeSts"
  LngHMI/4 -> Signal_CruiseChauffer_Sts/1  "Signal_CruiseChauffer_Sts"
  LngHMI/5 -> Signal_ACCTextDisp/1  "Signal_ACCTextDisp"
  LngHMI/6 -> Signal_TJATextDisp/1  "Signal_TJATextDisp"
  LngHMI/7 -> Signal_CCTextDisp/1  "Signal_CCTextDisp"
  LngHMI/8 -> Signal_HWAModeDisp/1  "Signal_HWAModeDisp"
  Constant/1 -> Bus Creator3/2  "LC_ReqUserConfirm"
  [ISL_ReqUserConfirm] -> Bus Creator3/1
  Bus Creator3/1 -> UOMSysFeedBack/1
  LngHMI/9 -> Signal_HWATextDisp/1  "Signal_HWATextDisp"
  [ACCFailure] -> Unit Delay/1
  HWA/12 -> [TJAActive]
  [TJAActive] -> Unit Delay1/1
  Unit Delay1/1 -> ACC/12
  Bus Selector8/21 -> HWA_AD/21  "<NOH_Swt_Req>"
  [AD_CAN] -> Bus Selector14/1
  Bus Selector14/1 -> SetSpd/17  "<DrvSBR>"
  Bus Selector14/2 -> SetSpd/18  "<PassSBR>"

== system PvtSubSys_VSM_ALL/Subsystem/StateManage/Enlong2s1/SignalRising ==
  In1 : Inport
  Relational Operator : RelationalOperator  Operator=>  OutDataTypeStr=boolean  RndMeth=Simplest
  Unit Delay : UnitDelay  SampleTime=-1  HasFrameUpgradeWarning=on
  Out1 : Outport
  wires:
  Unit Delay/1 -> Relational Operator/2
  Relational Operator/1 -> Out1/1
  In1/1 -> Unit Delay/1, Relational Operator/1
